simulink model "control"  (R2023a)
settings: Solver=VariableStepAuto  StartTime=0.0  StopTime=10.0  RelTol=1e-3
undefined symbols (not defined in the file or in its folder): desired_EMG, desired_wp
libraries: simulink x1, slpidlib x1
settings Model: Creator=s202421  LastModifiedBy=s202421

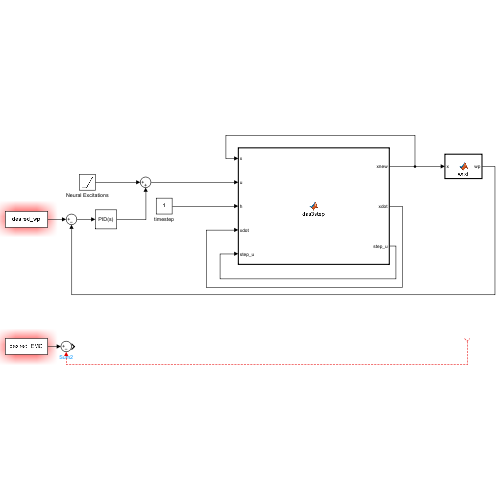
[thumbnail: Simulink's stored preview of the top-level diagram]
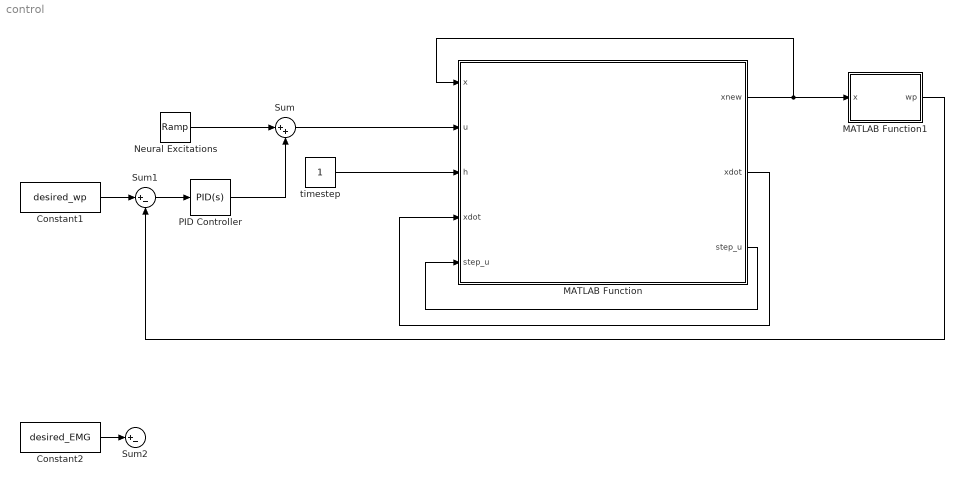
== system control ==
  Constant1 : Constant  Value=desired_wp
  Constant2 : Constant  Value=desired_EMG
  MATLAB Function : MATLAB Function  TreatAsAtomicUnit=on
  MATLAB Function1 : MATLAB Function  TreatAsAtomicUnit=on
  Neural Excitations : simulink/Sources/Ramp  slope=1  start=0  InitialOutput=0
  PID Controller : slpidlib/PID Controller  Controller=PID  Form=Parallel  TimeDomain=Continuous-time  UseExternalTs=off  SampleTime=-1  IntegratorMethod=Forward Euler  FilterMethod=Forward Euler  ControllerParametersSource=internal  P=1  I=1  UseKiTs=off  D=0  N=100  UseFilter=on  TunerSelectOption=Transfer Function Based (PID Tuner App)  InitialConditionSource=internal  InitialConditionForIntegrator=0  InitialConditionForFilter=0  DifferentiatorICPrevScaledInput=0  ExternalReset=none  TrackingMode=off  Kt=1  LimitOutput=off  SatLimitsSource=internal  UpperSaturationLimit=inf  LowerSaturationLimit=-inf  LinearizeAsGain=on  AntiWindupMode=none  Kb=1  LimitIntegrator=off  UpperIntegratorSaturationLimit=inf  LowerIntegratorSaturationLimit=-inf  POutMin=[]  POutMax=[]  IOutMin=[]  IOutMax=[]  DOutMin=[]  DOutMax=[]  NOutMin=[]  NOutMax=[]  SumOutMin=[]  SumOutMax=[]  SaturationOutMin=[]  SaturationOutMax=[]  PParamMin=[]  PParamMax=[]  IParamMin=[]  IParamMax=[]  DParamMin=[]  DParamMax=[]  NParamMin=[]  NParamMax=[]  KbParamMin=[]  KbParamMax=[]  KtParamMin=[]  KtParamMax=[]  KbOutMin=[]  KbOutMax=[]  KtOutMin=[]  KtOutMax=[]  IntegratorOutMin=[]  IntegratorOutMax=[]  FilterOutMin=[]  FilterOutMax=[]  SumI1OutMin=[]  SumI1OutMax=[]  SumI2OutMin=[]  SumI2OutMax=[]  SumI3OutMin=[]  SumI3OutMax=[]  SumI4OutMin=[]  SumI4OutMax=[]  SumDOutMin=[]  SumDOutMax=[]  DifferentiatorOutMin=[]  DifferentiatorOutMax=[]  FilterDiffOutCoefMin=[]  FilterDiffOutCoefMax=[]  ReciprocalOutMin=[]  ReciprocalOutMax=[]  SumDenOutMin=[]  SumDenOutMax=[]  SumNumOutMin=[]  SumNumOutMax=[]  DivideOutMin=[]  DivideOutMax=[]  UdiffTsProdOutMin=[]  UdiffTsProdOutMax=[]  NTsProdOutMin=[]  NTsProdOutMax=[]  UintegralTsProdOutMin=[]  UintegralTsProdOutMax=[]  UngainTsProdOutMin=[]  UngainTsProdOutMax=[]  ClampingZeroOutDataTypeStr=Inherit: Inherit via back propagation  ClampingZeroOutMin=[]  ClampingZeroOutMax=[]  FilterDenConstantOutDataTypeStr=Inherit: Inherit via back propagation  FilterDenConstantOutMin=[]  FilterDenConstantOutMax=[]  PCopyOutDataTypeStr=Inherit: Inherit via back propagation  PCopyOutMin=[]  PCopyOutMax=[]  NCopyOutDataTypeStr=Inherit: Inherit via back propagation  NCopyOutMin=[]  NCopyOutMax=[]  IntegratorContinuousStateAttributes=''  IntegratorStateMustResolveToSignalObject=off  IntegratorRTWStateStorageClass=Auto  FilterContinuousStateAttributes=''  FilterStateMustResolveToSignalObject=off  FilterRTWStateStorageClass=Auto  ParallelPVariant=InternalParameters  IdealPVariant=Disabled  IVariant=InternalParameters  DVariant=InternalParameters  IntegratorVariant=Continuous  SatVariant=Disabled  AWVariant=Passthrough  PCopyVariant=Disabled  TRVariant=Disabled  FdbkBlocksVariant=Forward  IdealPFdbkVariant=Disabled  SatFdbkVariant=Disabled  DerivativeFilterVariant=ContFilter  NVariant=InternalParameters  NCopyVariant=Disabled  FilterICVariant=InternalICsFilter  IntegratorICVariant=InternalICs  ExternalResetVariant=Disabled  TRSumVariant=Passthrough  SumFdbkVariant=Disabled  SumVariant=Sum_PID  TsampFilterVariant=InternalTs  TsampNgainVariant=Passthrough  TsampIntegralVariant=Passthrough  ExternalSaturationOutDataTypeStr=Inherit: Same as second input
  Sum : Sum  Inputs=|++
  Sum1 : Sum  Inputs=|+-
  Sum2 : Sum  Inputs=|+-
  timestep : Constant
  wires:
  MATLAB Function/2(xdot) -> MATLAB Function/4("xdot ")
  MATLAB Function/3(step_u) -> MATLAB Function/5("step_u ")
  MATLAB Function/1(xnew) -> MATLAB Function/1(x), MATLAB Function1/1(x)
  timestep/1 -> MATLAB Function/3(h)
  Neural Excitations/1 -> Sum/1
  Sum/1 -> MATLAB Function/2(u)
  MATLAB Function1/1(wp) -> Sum1/2
  Constant1/1 -> Sum1/1
  Sum1/1 -> PID Controller/1
  PID Controller/1 -> Sum/2
  Constant2/1 -> Sum2/1
  ? -> Sum2/2

== matlab function control/MATLAB Function1 ==
  data: x input; wp output
function wp = wrist(x)

y = u;

== matlab function control/MATLAB Function ==
  data: x input; u input; xnew output; h input; xdot input; step_u input; xdot output; step_u output
function [xnew, xdot, step_u]  = das3step(x, u, h, xdot, step_u)
	% Ton van den Bogert
	% (c) 2010-2011 Case Western Reserve University
    %
	% For dynamic simulation.  Advances the model by one time step.
    %
	% Inputs
	%	x		(298 x 1) System state
	%	u		(138 x 1) Muscle excitations, assumed constant during the time step
	%	h		(scalar)  Time step size
    %   xdot    (298 x 1) System state derivatives (initially zero)
	%	step_u	(138 x 1) Muscle excitations from previous step (initially zero)
    %
    % Optional inputs
    % 	M		(5 x 1)	  Moments applied to the thorax-humerus YZY axes and the elbow flexion and supination axes
	%   exF     (2 x 1)   Vertical force of amplitude exF(2) applied to the ulna at a distance of exF(1) from the elbow 
	%						(to simulate a mobile arm support)
    %   handF   (3 x 1)   Force at the CoM of the hand
    %
	% Outputs
	%	xnew	(298 x 1) The system state at the end of the time step
	%	FGH		(3 x 1)   The glenohumeral reaction force, acting on the scapula
    %
	% Method: First order Rosenbrock formula on implicit differential equation	
	
	% Evaluate dynamics in current x and xdot
    if nargin>7
        [f, dfdx, dfdxdot, dfdu, FGH] = das3('Dynamics',x,xdot,step_u,M,exF,handF);
    elseif nargin>6
        [f, dfdx, dfdxdot, dfdu, FGH] = das3('Dynamics',x,xdot,step_u,M,exF);
    elseif nargin>5
        [f, dfdx, dfdxdot, dfdu, FGH] = das3('Dynamics',x,xdot,step_u,M);
    else
        [f, dfdx, dfdxdot, dfdu, FGH] = das3('Dynamics',x,xdot,step_u);
    end
    
	% Solve the change in x from the 1st order Rosenbrock formula
	du = u - step_u;
	dx = (dfdx + dfdxdot/h)\(dfdxdot*xdot - f - dfdu*du);
	xnew = x + dx;
	
	% update variables for the next simulation step
	xdot = dx/h;
	step_u = u;


y = xnew;
